simulink model "sim_ballAndPlate"  (R2026a)
settings: Solver=FixedStepAuto  StopTime=inf  FixedStep=0.001
values from neighbouring files (symbols this model uses):
  g = 9.81    [MPC_design.m]
undefined symbols (not defined in the file or in its folder): I_max, x_init, x_max
libraries: slpidlib x2
settings Model: Creator=thoma  LastModifiedBy=alexi

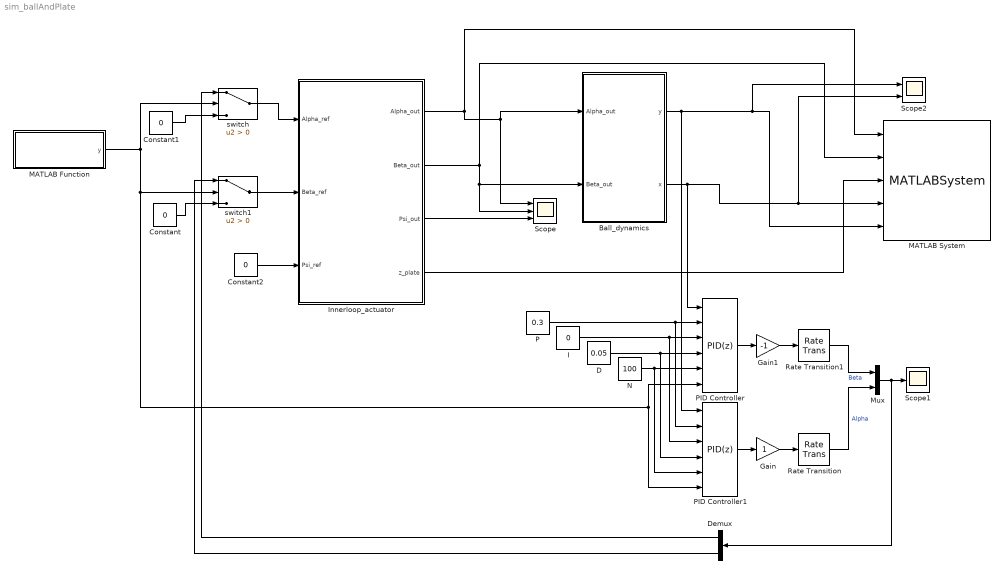
== system sim_ballAndPlate ==
  Ball_dynamics : Subsystem
  Constant : Constant  Value=0
  Constant1 : Constant  Value=0
  Constant2 : Constant  Value=0
  D : Constant  Value=0.05
  Demux : Demux  Outputs=2
  Gain : Gain
  Gain1 : Gain  Gain=-1
  I : Constant  Value=0
  Innerloop_actuator : Subsystem
  MATLAB Function : MATLAB Function  TreatAsAtomicUnit=on
  MATLAB System : MATLABSystem  System=PlateVisualizer  SimulateUsing=Code generation
      mask Type: PlateVisualizer
  Mux : Mux  Inputs=2
  N : Constant  Value=100
  P : Constant  Value=0.3
  PID Controller : slpidlib/PID Controller  Controller=PID  Form=Parallel  TimeDomain=Discrete-time  UseExternalTs=off  SampleTime=-1  IntegratorMethod=Forward Euler  FilterMethod=Forward Euler  ControllerParametersSource=external  P=1  I=1  UseKiTs=on  D=0  UseExternalDerivativeSource=off  N=100  UseFilter=on  TunerSelectOption=Transfer Function Based (PID Tuner App)  InitialConditionSource=internal  InitialConditionForIntegrator=0  InitialConditionForFilter=0  DifferentiatorICPrevScaledInput=0  ExternalReset=rising  TrackingMode=off  Kt=1  LimitOutput=off  SatLimitsSource=internal  UpperSaturationLimit=inf  LowerSaturationLimit=-inf  LinearizeAsGain=on  AntiWindupMode=none  Kb=1  LimitIntegrator=off  UpperIntegratorSaturationLimit=inf  LowerIntegratorSaturationLimit=-inf  POutMin=[]  POutMax=[]  IOutMin=[]  IOutMax=[]  DOutMin=[]  DOutMax=[]  NOutMin=[]  NOutMax=[]  SumOutMin=[]  SumOutMax=[]  SaturationOutMin=[]  SaturationOutMax=[]  PParamMin=[]  PParamMax=[]  IParamMin=[]  IParamMax=[]  DParamMin=[]  DParamMax=[]  NParamMin=[]  NParamMax=[]  KbParamMin=[]  KbParamMax=[]  KtParamMin=[]  KtParamMax=[]  KbOutMin=[]  KbOutMax=[]  KtOutMin=[]  KtOutMax=[]  IntegratorOutMin=[]  IntegratorOutMax=[]  FilterOutMin=[]  FilterOutMax=[]  SumI1OutMin=[]  SumI1OutMax=[]  SumI2OutMin=[]  SumI2OutMax=[]  SumI3OutMin=[]  SumI3OutMax=[]  SumI4OutMin=[]  SumI4OutMax=[]  SumDOutMin=[]  SumDOutMax=[]  DifferentiatorOutMin=[]  DifferentiatorOutMax=[]  FilterDiffOutCoefMin=[]  FilterDiffOutCoefMax=[]  ReciprocalOutMin=[]  ReciprocalOutMax=[]  SumDenOutMin=[]  SumDenOutMax=[]  SumNumOutMin=[]  SumNumOutMax=[]  DivideOutMin=[]  DivideOutMax=[]  UdiffTsProdOutMin=[]  UdiffTsProdOutMax=[]  NTsProdOutMin=[]  NTsProdOutMax=[]  UintegralTsProdOutMin=[]  UintegralTsProdOutMax=[]  UngainTsProdOutMin=[]  UngainTsProdOutMax=[]  ClampingZeroOutDataTypeStr=Inherit: Inherit via back propagation  ClampingZeroOutMin=[]  ClampingZeroOutMax=[]  FilterDenConstantOutDataTypeStr=Inherit: Inherit via back propagation  FilterDenConstantOutMin=[]  FilterDenConstantOutMax=[]  PCopyOutDataTypeStr=Inherit: Inherit via back propagation  PCopyOutMin=[]  PCopyOutMax=[]  NCopyOutDataTypeStr=Inherit: Inherit via back propagation  NCopyOutMin=[]  NCopyOutMax=[]  IntegratorContinuousStateAttributes=''  IntegratorStateMustResolveToSignalObject=off  IntegratorRTWStateStorageClass=Auto  FilterContinuousStateAttributes=''  FilterStateMustResolveToSignalObject=off  FilterRTWStateStorageClass=Auto  ParallelPVariant=ExternalParameters  IdealPVariant=Disabled  IVariant=ExternalParameters  DVariant=ExternalParameters  IntegratorVariant=Discrete  SatVariant=Disabled  AWVariant=Passthrough  PCopyVariant=Disabled  TRVariant=Disabled  FdbkBlocksVariant=Forward  IdealPFdbkVariant=Disabled  SatFdbkVariant=Disabled  DerivativeFilterVariant=ForwardEulerFilter  NVariant=ExternalParameters  NCopyVariant=Disabled  FilterICVariant=InternalICsFilter  IntegratorICVariant=InternalICs  ExternalResetVariant=ExternalReset  TRSumVariant=Passthrough  SumFdbkVariant=Disabled  SumVariant=Sum_PID  TsampFilterVariant=InternalTs  TsampNgainVariant=Passthrough  TsampIntegralVariant=Disabled_SignalSpec  ExternalSaturationOutDataTypeStr=Inherit: Same as second input  DerivativeSourceVariant=ErrorSignal  PreIntVariant=InternalPreInt
  PID Controller1 : slpidlib/PID Controller  Controller=PID  Form=Parallel  TimeDomain=Discrete-time  UseExternalTs=off  SampleTime=-1  IntegratorMethod=Forward Euler  FilterMethod=Forward Euler  ControllerParametersSource=external  P=1  I=1  UseKiTs=on  D=0  UseExternalDerivativeSource=off  N=100  UseFilter=on  TunerSelectOption=Transfer Function Based (PID Tuner App)  InitialConditionSource=internal  InitialConditionForIntegrator=0  InitialConditionForFilter=0  DifferentiatorICPrevScaledInput=0  ExternalReset=rising  TrackingMode=off  Kt=1  LimitOutput=off  SatLimitsSource=internal  UpperSaturationLimit=inf  LowerSaturationLimit=-inf  LinearizeAsGain=on  AntiWindupMode=none  Kb=1  LimitIntegrator=off  UpperIntegratorSaturationLimit=inf  LowerIntegratorSaturationLimit=-inf  POutMin=[]  POutMax=[]  IOutMin=[]  IOutMax=[]  DOutMin=[]  DOutMax=[]  NOutMin=[]  NOutMax=[]  SumOutMin=[]  SumOutMax=[]  SaturationOutMin=[]  SaturationOutMax=[]  PParamMin=[]  PParamMax=[]  IParamMin=[]  IParamMax=[]  DParamMin=[]  DParamMax=[]  NParamMin=[]  NParamMax=[]  KbParamMin=[]  KbParamMax=[]  KtParamMin=[]  KtParamMax=[]  KbOutMin=[]  KbOutMax=[]  KtOutMin=[]  KtOutMax=[]  IntegratorOutMin=[]  IntegratorOutMax=[]  FilterOutMin=[]  FilterOutMax=[]  SumI1OutMin=[]  SumI1OutMax=[]  SumI2OutMin=[]  SumI2OutMax=[]  SumI3OutMin=[]  SumI3OutMax=[]  SumI4OutMin=[]  SumI4OutMax=[]  SumDOutMin=[]  SumDOutMax=[]  DifferentiatorOutMin=[]  DifferentiatorOutMax=[]  FilterDiffOutCoefMin=[]  FilterDiffOutCoefMax=[]  ReciprocalOutMin=[]  ReciprocalOutMax=[]  SumDenOutMin=[]  SumDenOutMax=[]  SumNumOutMin=[]  SumNumOutMax=[]  DivideOutMin=[]  DivideOutMax=[]  UdiffTsProdOutMin=[]  UdiffTsProdOutMax=[]  NTsProdOutMin=[]  NTsProdOutMax=[]  UintegralTsProdOutMin=[]  UintegralTsProdOutMax=[]  UngainTsProdOutMin=[]  UngainTsProdOutMax=[]  ClampingZeroOutDataTypeStr=Inherit: Inherit via back propagation  ClampingZeroOutMin=[]  ClampingZeroOutMax=[]  FilterDenConstantOutDataTypeStr=Inherit: Inherit via back propagation  FilterDenConstantOutMin=[]  FilterDenConstantOutMax=[]  PCopyOutDataTypeStr=Inherit: Inherit via back propagation  PCopyOutMin=[]  PCopyOutMax=[]  NCopyOutDataTypeStr=Inherit: Inherit via back propagation  NCopyOutMin=[]  NCopyOutMax=[]  IntegratorContinuousStateAttributes=''  IntegratorStateMustResolveToSignalObject=off  IntegratorRTWStateStorageClass=Auto  FilterContinuousStateAttributes=''  FilterStateMustResolveToSignalObject=off  FilterRTWStateStorageClass=Auto  ParallelPVariant=ExternalParameters  IdealPVariant=Disabled  IVariant=ExternalParameters  DVariant=ExternalParameters  IntegratorVariant=Discrete  SatVariant=Disabled  AWVariant=Passthrough  PCopyVariant=Disabled  TRVariant=Disabled  FdbkBlocksVariant=Forward  IdealPFdbkVariant=Disabled  SatFdbkVariant=Disabled  DerivativeFilterVariant=ForwardEulerFilter  NVariant=ExternalParameters  NCopyVariant=Disabled  FilterICVariant=InternalICsFilter  IntegratorICVariant=InternalICs  ExternalResetVariant=ExternalReset  TRSumVariant=Passthrough  SumFdbkVariant=Disabled  SumVariant=Sum_PID  TsampFilterVariant=InternalTs  TsampNgainVariant=Passthrough  TsampIntegralVariant=Disabled_SignalSpec  ExternalSaturationOutDataTypeStr=Inherit: Same as second input  DerivativeSourceVariant=ErrorSignal  PreIntVariant=InternalPreInt
  Rate Transition : RateTransition
  Rate Transition1 : RateTransition
  Scope : Scope  NumInputPorts=3
      settings: ActiveDisplayYMinimum=-0.0096672380252072077  ActiveDisplayYMaximum=0.013010069028074875  DataLoggingVariableName=ScopeData2
  Scope1 : Scope
      settings: ActiveDisplayYMinimum=-0.047678013260338208  ActiveDisplayYMaximum=0.046983853602489342  DataLoggingVariableName=ScopeData6
  Scope2 : Scope  NumInputPorts=2
      settings: ActiveDisplayYMinimum=0.0046333567921488829  ActiveDisplayYMaximum=0.16615184924531679  DataLoggingVariableName=ScopeData7
  switch : Switch  Criteria=u2 > Threshold  SaturateOnIntegerOverflow=off  InputSameDT=off
  switch1 : Switch  Criteria=u2 > Threshold  SaturateOnIntegerOverflow=off  InputSameDT=off
  wires:
  Constant2/1 -> Innerloop_actuator/3(Psi_ref)
  Innerloop_actuator/2(Beta_out) -> Scope/2, Ball_dynamics/2(Beta_out), MATLAB System/2
  Innerloop_actuator/1(Alpha_out) -> Scope/1, Ball_dynamics/1(Alpha_out), MATLAB System/1
  Innerloop_actuator/3(Psi_out) -> Scope/3
  Ball_dynamics/1(y) -> PID Controller1/1, Scope2/1, MATLAB System/5
  Ball_dynamics/2(x) -> PID Controller/1, Scope2/2, MATLAB System/4
  MATLAB Function/1(y) -> switch/2, PID Controller1/6, PID Controller/6, switch1/2
  switch1/1 -> Innerloop_actuator/2(Beta_ref)
  switch/1 -> Innerloop_actuator/1(Alpha_ref)
  Innerloop_actuator/4(z_plate) -> MATLAB System/3
  PID Controller1/1 -> Gain/1
  Constant1/1 -> switch/3
  Constant/1 -> switch1/3
  N/1 -> PID Controller1/5, PID Controller/5
  D/1 -> PID Controller1/4, PID Controller/4
  I/1 -> PID Controller1/3, PID Controller/3
  P/1 -> PID Controller1/2, PID Controller/2
  PID Controller/1 -> Gain1/1
  Rate Transition1/1 -> Mux/1  "Beta"
  Rate Transition/1 -> Mux/2  "Alpha"
  Mux/1 -> Demux/1, Scope1/1
  Gain/1 -> Rate Transition/1
  Demux/1 -> switch/1
  Demux/2 -> switch1/1
  Gain1/1 -> Rate Transition1/1

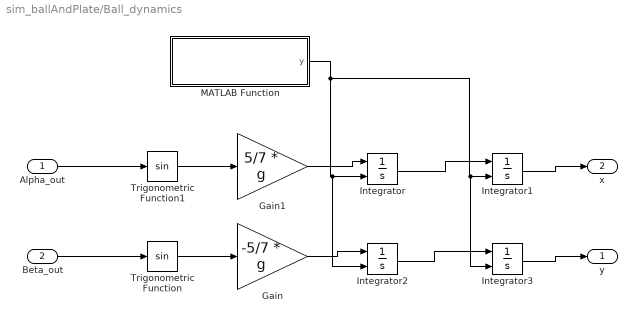
== system sim_ballAndPlate/Ball_dynamics ==
  Alpha_out : Inport
  Beta_out : Inport  Port=2
  Gain : Gain  Gain=-5/7 * g
  Gain1 : Gain  Gain=5/7 * g
  Integrator : Integrator  ExternalReset=rising
  Integrator1 : Integrator  ExternalReset=rising  InitialCondition=0.1
  Integrator2 : Integrator  ExternalReset=rising
  Integrator3 : Integrator  ExternalReset=rising  InitialCondition=0.15
  MATLAB Function : MATLAB Function  TreatAsAtomicUnit=on
  Trigonometric Function : Trigonometry
  Trigonometric Function1 : Trigonometry
  y : Outport
  x : Outport  Port=2
  wires:
  Beta_out/1 -> Trigonometric Function/1
  Trigonometric Function/1 -> Gain/1
  Gain/1 -> Integrator2/1
  Trigonometric Function1/1 -> Gain1/1
  Alpha_out/1 -> Trigonometric Function1/1
  Gain1/1 -> Integrator/1
  Integrator/1 -> Integrator1/1
  Integrator1/1 -> x/1
  Integrator2/1 -> Integrator3/1
  Integrator3/1 -> y/1
  MATLAB Function/1(y) -> Integrator3/2, Integrator1/2, Integrator2/2, Integrator/2

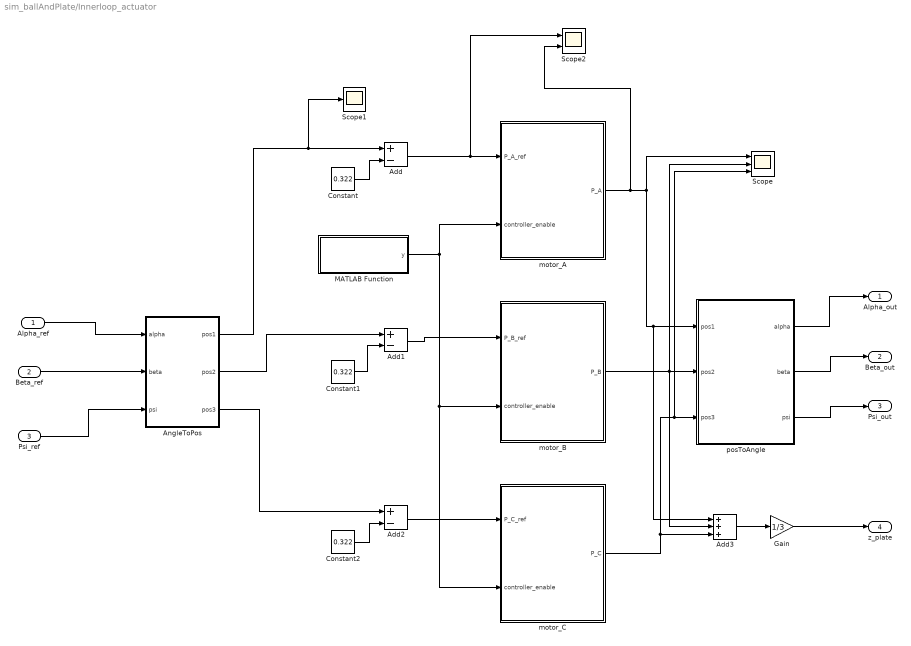
== system sim_ballAndPlate/Innerloop_actuator ==
  Alpha_ref : Inport
  Beta_ref : Inport  Port=2
  Psi_ref : Inport  Port=3
  Add : Sum  Inputs=+-
  Add1 : Sum  Inputs=+-
  Add2 : Sum  Inputs=+-
  Add3 : Sum  Inputs=+++
  "AngleToPos " : MATLAB Function  TreatAsAtomicUnit=on
  Constant : Constant  Value=0.322
  Constant1 : Constant  Value=0.322
  Constant2 : Constant  Value=0.322
  Gain : Gain  Gain=1/3
  MATLAB Function : MATLAB Function  TreatAsAtomicUnit=on
  Scope : Scope  NumInputPorts=3
      settings: ActiveDisplayYMinimum=-0.024286894583428403  ActiveDisplayYMaximum=0.0026985438426031555
  Scope1 : Scope
      settings: ActiveDisplayYMinimum=0.3217331997726901  ActiveDisplayYMaximum=0.32218451733100706
  Scope2 : Scope  NumInputPorts=2
      settings: ActiveDisplayYMinimum=-0.024653412981581042  ActiveDisplayYMaximum=0.021597858954205081  DataLoggingVariableName=ScopeData4
  motor_A : Subsystem
  motor_B : Subsystem
  motor_C : Subsystem
  posToAngle : MATLAB Function  TreatAsAtomicUnit=on
  Alpha_out : Outport
  Beta_out : Outport  Port=2
  Psi_out : Outport  Port=3
  z_plate : Outport  Port=4
  wires:
  Alpha_ref/1 -> "AngleToPos "/1(alpha)
  Beta_ref/1 -> "AngleToPos "/2(beta)
  Psi_ref/1 -> "AngleToPos "/3(psi)
  Constant/1 -> Add/2
  Add/1 -> Scope2/1, motor_A/1(P_A_ref)
  motor_A/1(P_A) -> Scope2/2, Add3/1, posToAngle/1(pos1), Scope/1
  "AngleToPos "/1(pos1) -> Scope1/1, Add/1
  posToAngle/1(alpha) -> Alpha_out/1
  "AngleToPos "/2(pos2) -> Add1/1
  Add1/1 -> motor_B/1(P_B_ref)
  Constant1/1 -> Add1/2
  "AngleToPos "/3(pos3) -> Add2/1
  Add2/1 -> motor_C/1(P_C_ref)
  Constant2/1 -> Add2/2
  motor_C/1(P_C) -> Add3/3, Scope/3, posToAngle/3(pos3)
  motor_B/1(P_B) -> Scope/2, posToAngle/2(pos2), Add3/2
  posToAngle/2(beta) -> Beta_out/1
  posToAngle/3(psi) -> Psi_out/1
  MATLAB Function/1(y) -> motor_C/2(controller_enable), motor_B/2(controller_enable), motor_A/2(controller_enable)
  Add3/1 -> Gain/1
  Gain/1 -> z_plate/1

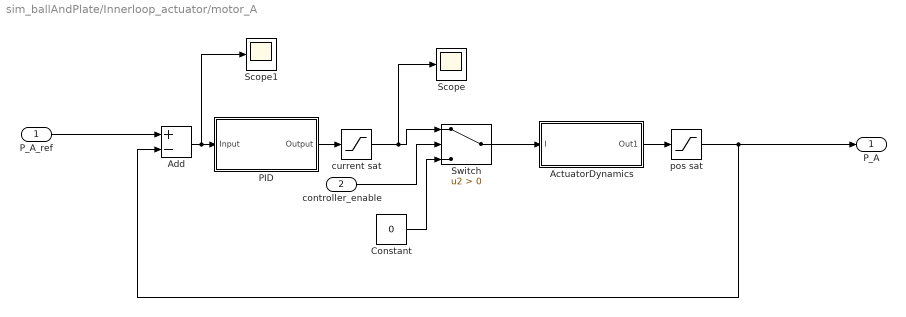
== system sim_ballAndPlate/Innerloop_actuator/motor_A ==
  P_A_ref : Inport
  controller_enable : Inport  Port=2
  ActuatorDynamics : Subsystem
  Add : Sum  Inputs=+-
  Constant : Constant  Value=0
  PID : Subsystem
  Scope : Scope
      settings: ActiveDisplayYMinimum=-0.2151003532733422  ActiveDisplayYMaximum=0.78783772218945147  DataLoggingVariableName=ScopeData3
  Scope1 : Scope
      settings: ActiveDisplayYMinimum=-0.013802200769437761  ActiveDisplayYMaximum=0.022158674956348122  DataLoggingVariableName=ScopeData5
  Switch : Switch  Criteria=u2 > Threshold  SaturateOnIntegerOverflow=off  InputSameDT=off
  current sat : Saturate  UpperLimit=I_max  LowerLimit=-I_max
  pos sat : Saturate  UpperLimit=x_max  LowerLimit=-x_max
  P_A : Outport
  wires:
  P_A_ref/1 -> Add/1
  PID/1(Output) -> current sat/1
  ActuatorDynamics/1(Out1) -> pos sat/1
  pos sat/1 -> Add/2, P_A/1
  controller_enable/1 -> Switch/2
  current sat/1 -> Scope/1, Switch/1
  Switch/1 -> ActuatorDynamics/1(I)
  Constant/1 -> Switch/3
  Add/1 -> Scope1/1, PID/1(Input)

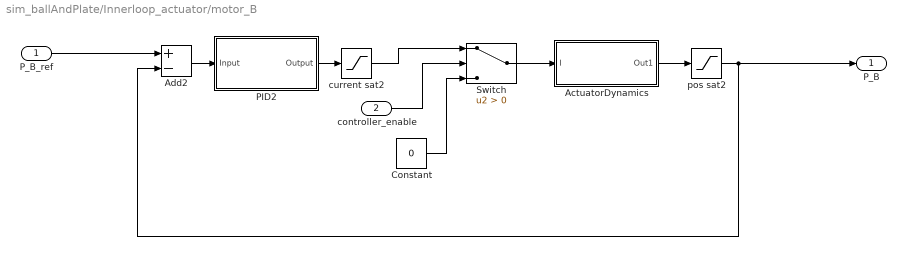
== system sim_ballAndPlate/Innerloop_actuator/motor_B ==
  P_B_ref : Inport
  controller_enable : Inport  Port=2
  ActuatorDynamics : Subsystem
  Add2 : Sum  Inputs=+-
  Constant : Constant  Value=0
  PID2 : Subsystem
  Switch : Switch  Criteria=u2 > Threshold  SaturateOnIntegerOverflow=off  InputSameDT=off
  current sat2 : Saturate  UpperLimit=I_max  LowerLimit=-I_max
  pos sat2 : Saturate  UpperLimit=x_max  LowerLimit=-x_max
  P_B : Outport
  wires:
  controller_enable/1 -> Switch/2
  Switch/1 -> ActuatorDynamics/1(I)
  ActuatorDynamics/1(Out1) -> pos sat2/1
  P_B_ref/1 -> Add2/1
  pos sat2/1 -> Add2/2, P_B/1
  Add2/1 -> PID2/1(Input)
  PID2/1(Output) -> current sat2/1
  current sat2/1 -> Switch/1
  Constant/1 -> Switch/3

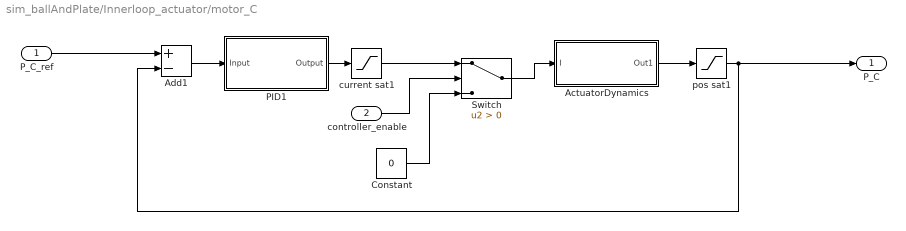
== system sim_ballAndPlate/Innerloop_actuator/motor_C ==
  P_C_ref : Inport
  controller_enable : Inport  Port=2
  ActuatorDynamics : Subsystem
  Add1 : Sum  Inputs=+-
  Constant : Constant  Value=0
  PID1 : Subsystem
  Switch : Switch  Criteria=u2 > Threshold  SaturateOnIntegerOverflow=off  InputSameDT=off
  current sat1 : Saturate  UpperLimit=I_max  LowerLimit=-I_max
  pos sat1 : Saturate  UpperLimit=x_max  LowerLimit=-x_max
  P_C : Outport
  wires:
  controller_enable/1 -> Switch/2
  Switch/1 -> ActuatorDynamics/1(I)
  ActuatorDynamics/1(Out1) -> pos sat1/1
  P_C_ref/1 -> Add1/1
  pos sat1/1 -> Add1/2, P_C/1
  Add1/1 -> PID1/1(Input)
  PID1/1(Output) -> current sat1/1
  current sat1/1 -> Switch/1
  Constant/1 -> Switch/3

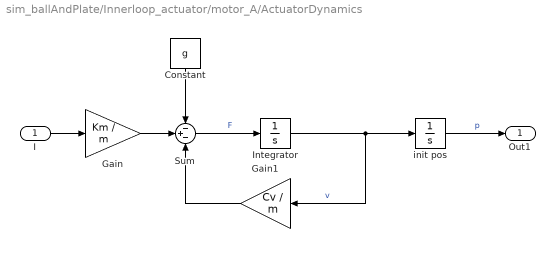
== system sim_ballAndPlate/Innerloop_actuator/motor_A/ActuatorDynamics ==
  I : Inport
  Constant : Constant  Value=g
  Gain : Gain  Gain=Km / m
  Gain1 : Gain  Gain=Cv / m
  Integrator : Integrator
  Sum : Sum  Inputs=-+-
  init pos : Integrator  InitialCondition=x_init
  Out1 : Outport
  wires:
  I/1 -> Gain/1
  Gain/1 -> Sum/2
  init pos/1 -> Out1/1  "p"
  Sum/1 -> Integrator/1  "F"
  Integrator/1 -> Gain1/1, init pos/1  "v"
  Gain1/1 -> Sum/3
  Constant/1 -> Sum/1

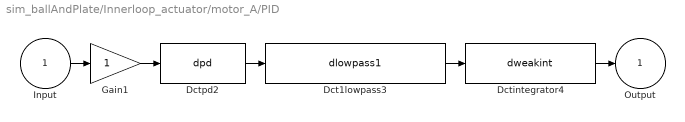
== system sim_ballAndPlate/Innerloop_actuator/motor_A/PID ==
  Input : Inport
  Dct1lowpass3 : S-Function  FunctionName=dlowpass1  Parameters=f_den, 0.001  SFunctionDeploymentMode=off  EnableBusSupport=off  mask(dctools){f_den=200}
      mask prompts: f_den "Pole [Hz]"
      mask help: This block implements a discrete time 1st order lowpass filter.
      mask Display: disp('DCT 1st order lowpass')
  Dctintegrator4 : S-Function  FunctionName=dweakint  Parameters=f_num, 0.001  SFunctionDeploymentMode=off  EnableBusSupport=off  mask(dctools){f_num=1}
      mask prompts: f_num "Zero [Hz]"
      mask help: This block implements a discrete time weak integrator filter.
      mask Display: disp('DCT integrator')
  Dctpd2 : S-Function  FunctionName=dpd  Parameters=kp, kv, 0.001  SFunctionDeploymentMode=off  EnableBusSupport=off  mask(dctools){kp=0.01, kv=10}
      mask help: This block implements a discrete time pd filter.
      mask Display: disp('DCT pd')
  Gain1 : Gain
  Output : Outport
  wires:
  Input/1 -> Gain1/1
  Gain1/1 -> Dctpd2/1
  Dctpd2/1 -> Dct1lowpass3/1
  Dct1lowpass3/1 -> Dctintegrator4/1
  Dctintegrator4/1 -> Output/1

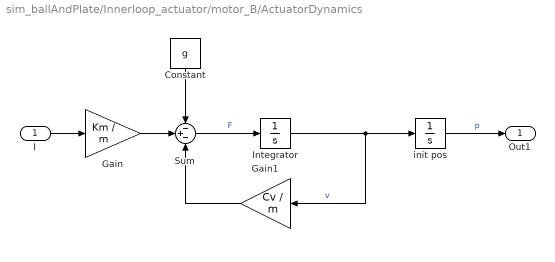
== system sim_ballAndPlate/Innerloop_actuator/motor_B/ActuatorDynamics ==
  I : Inport
  Constant : Constant  Value=g
  Gain : Gain  Gain=Km / m
  Gain1 : Gain  Gain=Cv / m
  Integrator : Integrator
  Sum : Sum  Inputs=-+-
  init pos : Integrator  InitialCondition=x_init
  Out1 : Outport
  wires:
  I/1 -> Gain/1
  Gain/1 -> Sum/2
  init pos/1 -> Out1/1  "p"
  Sum/1 -> Integrator/1  "F"
  Integrator/1 -> Gain1/1, init pos/1  "v"
  Gain1/1 -> Sum/3
  Constant/1 -> Sum/1

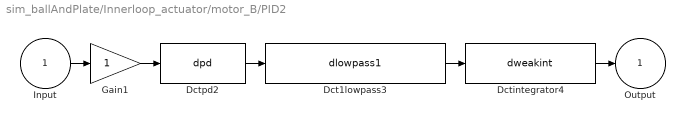
== system sim_ballAndPlate/Innerloop_actuator/motor_B/PID2 ==
  Input : Inport
  Dct1lowpass3 : S-Function  FunctionName=dlowpass1  Parameters=f_den, 0.001  SFunctionDeploymentMode=off  EnableBusSupport=off  mask(dctools){f_den=200}
      mask prompts: f_den "Pole [Hz]"
      mask help: This block implements a discrete time 1st order lowpass filter.
      mask Display: disp('DCT 1st order lowpass')
  Dctintegrator4 : S-Function  FunctionName=dweakint  Parameters=f_num, 0.001  SFunctionDeploymentMode=off  EnableBusSupport=off  mask(dctools){f_num=1}
      mask prompts: f_num "Zero [Hz]"
      mask help: This block implements a discrete time weak integrator filter.
      mask Display: disp('DCT integrator')
  Dctpd2 : S-Function  FunctionName=dpd  Parameters=kp, kv, 0.001  SFunctionDeploymentMode=off  EnableBusSupport=off  mask(dctools){kp=0.01, kv=10}
      mask help: This block implements a discrete time pd filter.
      mask Display: disp('DCT pd')
  Gain1 : Gain
  Output : Outport
  wires:
  Input/1 -> Gain1/1
  Gain1/1 -> Dctpd2/1
  Dctpd2/1 -> Dct1lowpass3/1
  Dct1lowpass3/1 -> Dctintegrator4/1
  Dctintegrator4/1 -> Output/1

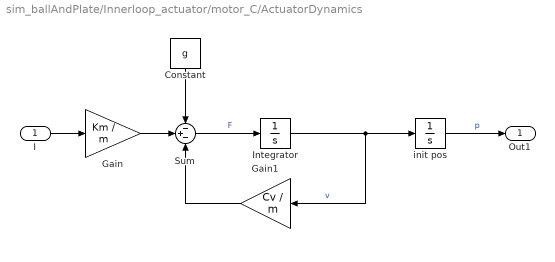
== system sim_ballAndPlate/Innerloop_actuator/motor_C/ActuatorDynamics ==
  I : Inport
  Constant : Constant  Value=g
  Gain : Gain  Gain=Km / m
  Gain1 : Gain  Gain=Cv / m
  Integrator : Integrator
  Sum : Sum  Inputs=-+-
  init pos : Integrator  InitialCondition=x_init
  Out1 : Outport
  wires:
  I/1 -> Gain/1
  Gain/1 -> Sum/2
  init pos/1 -> Out1/1  "p"
  Sum/1 -> Integrator/1  "F"
  Integrator/1 -> Gain1/1, init pos/1  "v"
  Gain1/1 -> Sum/3
  Constant/1 -> Sum/1

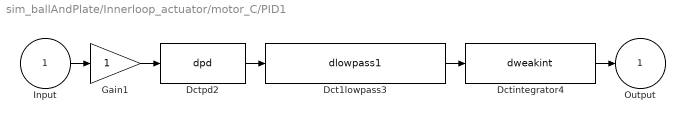
== system sim_ballAndPlate/Innerloop_actuator/motor_C/PID1 ==
  Input : Inport
  Dct1lowpass3 : S-Function  FunctionName=dlowpass1  Parameters=f_den, 0.001  SFunctionDeploymentMode=off  EnableBusSupport=off  mask(dctools){f_den=200}
      mask prompts: f_den "Pole [Hz]"
      mask help: This block implements a discrete time 1st order lowpass filter.
      mask Display: disp('DCT 1st order lowpass')
  Dctintegrator4 : S-Function  FunctionName=dweakint  Parameters=f_num, 0.001  SFunctionDeploymentMode=off  EnableBusSupport=off  mask(dctools){f_num=1}
      mask prompts: f_num "Zero [Hz]"
      mask help: This block implements a discrete time weak integrator filter.
      mask Display: disp('DCT integrator')
  Dctpd2 : S-Function  FunctionName=dpd  Parameters=kp, kv, 0.001  SFunctionDeploymentMode=off  EnableBusSupport=off  mask(dctools){kp=0.01, kv=10}
      mask help: This block implements a discrete time pd filter.
      mask Display: disp('DCT pd')
  Gain1 : Gain
  Output : Outport
  wires:
  Input/1 -> Gain1/1
  Gain1/1 -> Dctpd2/1
  Dctpd2/1 -> Dct1lowpass3/1
  Dct1lowpass3/1 -> Dctintegrator4/1
  Dctintegrator4/1 -> Output/1

== matlab function sim_ballAndPlate/MATLAB Function ==
  data: y output
function y = get_outer_loop_state()
    % This block queries the base workspace live at every single sample step
    % We declare evalin as extrinsic so the code generator bypasses it
    coder.extrinsic('evalin');
    
    % Initialize a safe compiled default value
    state_val = 0.0; 
    
    % Safely read the value from the MATLAB base workspace
    state_val = evalin('base', 'outer_loop_enable');
    
    % Cast the value to a standard double output
    y = double(state_val);
end

== matlab function sim_ballAndPlate/Innerloop_actuator/posToAngle ==
  data: pos1 input; alpha output; pos2 input; pos3 input; beta output; psi output
function [alpha, beta, psi] = posToAngle(pos1, pos2, pos3)
    % Returns the angles resulting from the given position
    % note: the position should be relative from the actuators midpoint in the global frame

    % Physical Constants
    r = 0.17;                 % Radius to joints (m)
    T = 0.322;                % Resting height (m)
    theta = deg2rad(120);     % angle between bases (rad)

    % Reconstruction of the Plate Unit Vectors 
    % We find where the joints are in the world frame by using the inputs
    % If pos = 0.322, the joints are exactly T_height above the base.
    P1_global = [r; 0; T + pos1];
    P2_global = [r*cos(theta); r*sin(theta); T + pos2];
    P3_global = [r*cos(theta); -r*sin(theta); T + pos3];

    % Find the center of the tilted plate
    % The average of the three joint positions gives the center of the motion plate
    center = (P1_global + P2_global + P3_global) / 3;

    % Vectors from the plate center to the joints
    % This isolates the tilt of the plate surface
    v1 = P1_global - center;
    v2 = P2_global - center;
    v3 = P3_global - center;

    % Compute Unit Vectors
    uX = v1 / norm(v1);             % Plate X-axis
    u_temp = cross(uX, v3);         % Temporary vector to find normal
    uZ = u_temp / norm(u_temp);     % Plate Z-axis (Normal)
    uY = cross(uZ, uX);             % Plate Y-axis

    % Extract Tait-Bryan Angles
    beta = asin(-uX(3));                            
    alpha = asin(uY(3) / sqrt(1 - uX(3)^2));       
    psi = asin(uX(2) / sqrt(1 - uX(3)^2));
end

== matlab function sim_ballAndPlate/Innerloop_actuator/MATLAB Function ==
  data: y output
function y = get_inner_loop_state()
    % This block queries the base workspace live at every single sample step
    % We declare evalin as extrinsic so the code generator bypasses it
    coder.extrinsic('evalin');
    
    % Initialize a safe compiled default value
    state_val = 0.0; 
    
    % Safely read the value from the MATLAB base workspace
    state_val = evalin('base', 'inner_loop_enable');
    
    % Cast the value to a standard double output
    y = double(state_val);
end

== matlab function sim_ballAndPlate/Ball_dynamics/MATLAB Function ==
  data: y output
function y = get_sim_reset_loop_state()
    % This block queries the base workspace live at every single sample step
    % We declare evalin as extrinsic so the code generator bypasses it
    coder.extrinsic('evalin');
    
    % Initialize a safe compiled default value
    state_val = 0.0; 
    
    % Safely read the value from the MATLAB base workspace
    state_val = evalin('base', 'sim_reset');
    
    % Cast the value to a standard double output
    y = double(state_val);
end

== matlab function sim_ballAndPlate/Innerloop_actuator/AngleToPos  ==
  data: alpha input; pos1 output; beta input; psi input; pos2 output; pos3 output
function [pos1, pos2, pos3] = angleToPos(alpha, beta, psi)
    % Returns the actuator positions required to reach the desired angle
    % note: the position is absolute in the global frame

    % Physical Constants
    r = 0.17;           % Joint radius (m)
    T = [0; 0; 0.322];  % Resting height vector (m)
    
    % Joint positions on base and plate (equilateral triangle)
    % These match the definitions in your posToAngle function
    theta = [0, deg2rad(240), deg2rad(120)];
    B = [r*cos(theta); r*sin(theta); zeros(1,3)]; % Base joints (b_i)
    P = [r*cos(theta); r*sin(theta); zeros(1,3)]; % Plate joints (p_i)
    
    % Rotation Matrices (Yaw-Pitch-Roll order)
    Rz = [cos(psi) -sin(psi) 0; sin(psi) cos(psi) 0; 0 0 1];
    Ry = [cos(beta) 0 sin(beta); 0 1 0; -sin(beta) 0 cos(beta)];
    Rx = [1 0 0; 0 cos(alpha) -sin(alpha); 0 sin(alpha) cos(alpha)];
    R_BtoP = Rz * Ry * Rx; 
    
    % Compute absolute position for each motor
    % Motor 1
    l1_vec = T + (R_BtoP * P(:,1)) - B(:,1);
    pos1 = norm(l1_vec);
    
    % Motor 2
    l2_vec = T + (R_BtoP * P(:,2)) - B(:,2);
    pos2 = norm(l2_vec);
    
    % Motor 3
    l3_vec = T + (R_BtoP * P(:,3)) - B(:,3);
    pos3 = norm(l3_vec);
end
